simulink model "PI_with_st_pttracking"  (R2021a)
settings: Solver=VariableStepAuto  StartTime=0.0  StopTime=2500  RelTol=1e-3
libraries: simulink x4, pid_lib x4
settings Model: Creator=jessilbijou  LastModifiedBy=jessilbijou

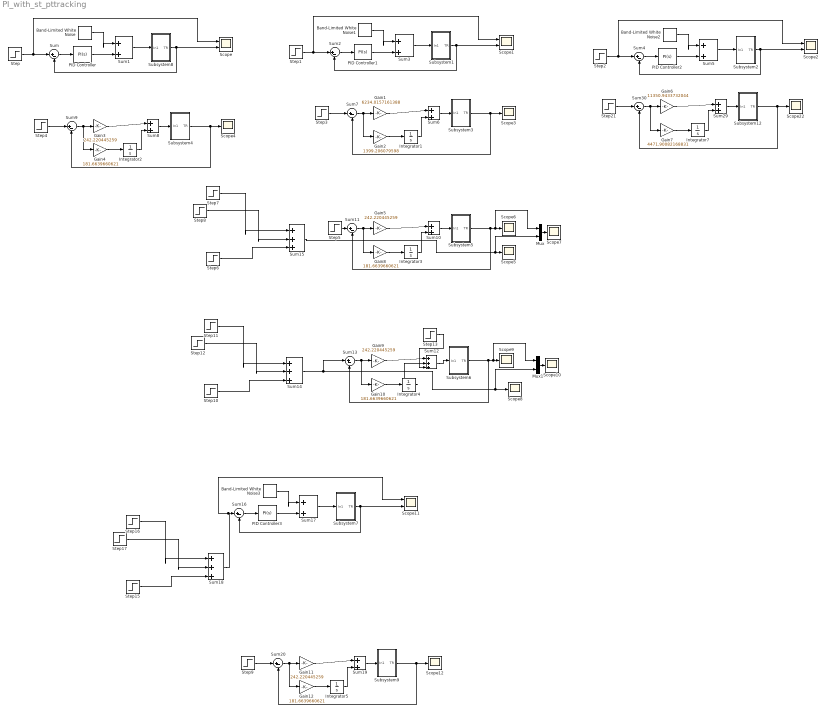
== system PI_with_st_pttracking ==
  Band-Limited White Noise{,1..3} (4 alike) : simulink/Sources/Band-Limited White Noise  Cov=[0.1]  Ts=0.1  seed=[23341]
  Gain1 : Gain  Gain=6234.0157161388
  Gain{4,8,10,12} (4 alike) : Gain  Gain=181.6639660621
  Gain{3,5,9,11} (4 alike) : Gain  Gain=242.220445259
  Gain2 : Gain  Gain=1399.206079598
  Gain6 : Gain  Gain=11350.9433732044
  Gain7 : Gain  Gain=4471.90082168831
  Integrator{1..5,7} (6 alike) : Integrator
  Mux : Mux  Inputs=2
  Mux1 : Mux  Inputs=2
  PID Controller : pid_lib/PID Controller  Controller=PI  Form=Parallel  TimeDomain=Continuous-time  UseExternalTs=off  SampleTime=-1  IntegratorMethod=Forward Euler  FilterMethod=Forward Euler  ControllerParametersSource=internal  P=242.220445259  I=181.6639660621  D=0  UseFilter=on  N=100  TunerSelectOption=Transfer Function Based (PID Tuner App)  InitialConditionSource=internal  InitialConditionForIntegrator=0  InitialConditionForFilter=0  DifferentiatorICPrevScaledInput=0  ExternalReset=none  TrackingMode=off  Kt=1  LimitOutput=off  SatLimitsSource=internal  UpperSaturationLimit=inf  LowerSaturationLimit=-inf  LinearizeAsGain=on  AntiWindupMode=none  Kb=1  POutMin=[]  POutMax=[]  IOutMin=[]  IOutMax=[]  DOutMin=[]  DOutMax=[]  NOutMin=[]  NOutMax=[]  SumOutMin=[]  SumOutMax=[]  SaturationOutMin=[]  SaturationOutMax=[]  PParamMin=[]  PParamMax=[]  IParamMin=[]  IParamMax=[]  DParamMin=[]  DParamMax=[]  NParamMin=[]  NParamMax=[]  KbParamMin=[]  KbParamMax=[]  KtParamMin=[]  KtParamMax=[]  KbOutMin=[]  KbOutMax=[]  KtOutMin=[]  KtOutMax=[]  IntegratorOutMin=[]  IntegratorOutMax=[]  FilterOutMin=[]  FilterOutMax=[]  SumI1OutMin=[]  SumI1OutMax=[]  SumI2OutMin=[]  SumI2OutMax=[]  SumI3OutMin=[]  SumI3OutMax=[]  SumI4OutMin=[]  SumI4OutMax=[]  SumDOutMin=[]  SumDOutMax=[]  DifferentiatorOutMin=[]  DifferentiatorOutMax=[]  FilterDiffOutCoefMin=[]  FilterDiffOutCoefMax=[]  ReciprocalOutMin=[]  ReciprocalOutMax=[]  SumDenOutMin=[]  SumDenOutMax=[]  SumNumOutMin=[]  SumNumOutMax=[]  DivideOutMin=[]  DivideOutMax=[]  UdiffTsProdOutMin=[]  UdiffTsProdOutMax=[]  NTsProdOutMin=[]  NTsProdOutMax=[]  UintegralTsProdOutMin=[]  UintegralTsProdOutMax=[]  UngainTsProdOutMin=[]  UngainTsProdOutMax=[]  IntegratorContinuousStateAttributes=''  IntegratorStateMustResolveToSignalObject=off  IntegratorRTWStateStorageClass=Auto  FilterContinuousStateAttributes=''  FilterStateMustResolveToSignalObject=off  FilterRTWStateStorageClass=Auto  ParallelPVariant=InternalParameters  IdealPVariant=Disabled  IVariant=InternalParameters  DVariant=Disabled  IntegratorVariant=Continuous  SatVariant=Disabled  AWVariant=Passthrough  PCopyVariant=Disabled  TRVariant=Disabled  FdbkBlocksVariant=Forward  IdealPFdbkVariant=Disabled  SatFdbkVariant=Disabled  DerivativeFilterVariant=Disabled  NVariant=Disabled  NCopyVariant=Disabled_SignalSpec  FilterICVariant=Disabled  IntegratorICVariant=InternalICs  ExternalResetVariant=Disabled  TRSumVariant=Passthrough  SumFdbkVariant=Disabled  SumVariant=Sum_PI  TsampFilterVariant=InternalTs  TsampNgainVariant=Passthrough  TsampIntegralVariant=Passthrough  ExternalSaturationOutDataTypeStr=Inherit: Same as second input
  PID Controller1 : pid_lib/PID Controller  Controller=PI  Form=Parallel  TimeDomain=Continuous-time  UseExternalTs=off  SampleTime=-1  IntegratorMethod=Forward Euler  FilterMethod=Forward Euler  ControllerParametersSource=internal  P=6234.0157161388  I=1399.206079598  D=0  UseFilter=on  N=100  TunerSelectOption=Transfer Function Based (PID Tuner App)  InitialConditionSource=internal  InitialConditionForIntegrator=0  InitialConditionForFilter=0  DifferentiatorICPrevScaledInput=0  ExternalReset=none  TrackingMode=off  Kt=1  LimitOutput=off  SatLimitsSource=internal  UpperSaturationLimit=inf  LowerSaturationLimit=-inf  LinearizeAsGain=on  AntiWindupMode=none  Kb=1  POutMin=[]  POutMax=[]  IOutMin=[]  IOutMax=[]  DOutMin=[]  DOutMax=[]  NOutMin=[]  NOutMax=[]  SumOutMin=[]  SumOutMax=[]  SaturationOutMin=[]  SaturationOutMax=[]  PParamMin=[]  PParamMax=[]  IParamMin=[]  IParamMax=[]  DParamMin=[]  DParamMax=[]  NParamMin=[]  NParamMax=[]  KbParamMin=[]  KbParamMax=[]  KtParamMin=[]  KtParamMax=[]  KbOutMin=[]  KbOutMax=[]  KtOutMin=[]  KtOutMax=[]  IntegratorOutMin=[]  IntegratorOutMax=[]  FilterOutMin=[]  FilterOutMax=[]  SumI1OutMin=[]  SumI1OutMax=[]  SumI2OutMin=[]  SumI2OutMax=[]  SumI3OutMin=[]  SumI3OutMax=[]  SumI4OutMin=[]  SumI4OutMax=[]  SumDOutMin=[]  SumDOutMax=[]  DifferentiatorOutMin=[]  DifferentiatorOutMax=[]  FilterDiffOutCoefMin=[]  FilterDiffOutCoefMax=[]  ReciprocalOutMin=[]  ReciprocalOutMax=[]  SumDenOutMin=[]  SumDenOutMax=[]  SumNumOutMin=[]  SumNumOutMax=[]  DivideOutMin=[]  DivideOutMax=[]  UdiffTsProdOutMin=[]  UdiffTsProdOutMax=[]  NTsProdOutMin=[]  NTsProdOutMax=[]  UintegralTsProdOutMin=[]  UintegralTsProdOutMax=[]  UngainTsProdOutMin=[]  UngainTsProdOutMax=[]  IntegratorContinuousStateAttributes=''  IntegratorStateMustResolveToSignalObject=off  IntegratorRTWStateStorageClass=Auto  FilterContinuousStateAttributes=''  FilterStateMustResolveToSignalObject=off  FilterRTWStateStorageClass=Auto  ParallelPVariant=InternalParameters  IdealPVariant=Disabled  IVariant=InternalParameters  DVariant=Disabled  IntegratorVariant=Continuous  SatVariant=Disabled  AWVariant=Passthrough  PCopyVariant=Disabled  TRVariant=Disabled  FdbkBlocksVariant=Forward  IdealPFdbkVariant=Disabled  SatFdbkVariant=Disabled  DerivativeFilterVariant=Disabled  NVariant=Disabled  NCopyVariant=Disabled_SignalSpec  FilterICVariant=Disabled  IntegratorICVariant=InternalICs  ExternalResetVariant=Disabled  TRSumVariant=Passthrough  SumFdbkVariant=Disabled  SumVariant=Sum_PI  TsampFilterVariant=InternalTs  TsampNgainVariant=Passthrough  TsampIntegralVariant=Passthrough  ExternalSaturationOutDataTypeStr=Inherit: Same as second input
  PID Controller2 : pid_lib/PID Controller  Controller=PI  Form=Parallel  TimeDomain=Continuous-time  UseExternalTs=off  SampleTime=-1  IntegratorMethod=Forward Euler  FilterMethod=Forward Euler  ControllerParametersSource=internal  P=11350.9433732044  I=4471.90082168831  D=0  UseFilter=on  N=100  TunerSelectOption=Transfer Function Based (PID Tuner App)  InitialConditionSource=internal  InitialConditionForIntegrator=0  InitialConditionForFilter=0  DifferentiatorICPrevScaledInput=0  ExternalReset=none  TrackingMode=off  Kt=1  LimitOutput=off  SatLimitsSource=internal  UpperSaturationLimit=inf  LowerSaturationLimit=-inf  LinearizeAsGain=on  AntiWindupMode=none  Kb=1  POutMin=[]  POutMax=[]  IOutMin=[]  IOutMax=[]  DOutMin=[]  DOutMax=[]  NOutMin=[]  NOutMax=[]  SumOutMin=[]  SumOutMax=[]  SaturationOutMin=[]  SaturationOutMax=[]  PParamMin=[]  PParamMax=[]  IParamMin=[]  IParamMax=[]  DParamMin=[]  DParamMax=[]  NParamMin=[]  NParamMax=[]  KbParamMin=[]  KbParamMax=[]  KtParamMin=[]  KtParamMax=[]  KbOutMin=[]  KbOutMax=[]  KtOutMin=[]  KtOutMax=[]  IntegratorOutMin=[]  IntegratorOutMax=[]  FilterOutMin=[]  FilterOutMax=[]  SumI1OutMin=[]  SumI1OutMax=[]  SumI2OutMin=[]  SumI2OutMax=[]  SumI3OutMin=[]  SumI3OutMax=[]  SumI4OutMin=[]  SumI4OutMax=[]  SumDOutMin=[]  SumDOutMax=[]  DifferentiatorOutMin=[]  DifferentiatorOutMax=[]  FilterDiffOutCoefMin=[]  FilterDiffOutCoefMax=[]  ReciprocalOutMin=[]  ReciprocalOutMax=[]  SumDenOutMin=[]  SumDenOutMax=[]  SumNumOutMin=[]  SumNumOutMax=[]  DivideOutMin=[]  DivideOutMax=[]  UdiffTsProdOutMin=[]  UdiffTsProdOutMax=[]  NTsProdOutMin=[]  NTsProdOutMax=[]  UintegralTsProdOutMin=[]  UintegralTsProdOutMax=[]  UngainTsProdOutMin=[]  UngainTsProdOutMax=[]  IntegratorContinuousStateAttributes=''  IntegratorStateMustResolveToSignalObject=off  IntegratorRTWStateStorageClass=Auto  FilterContinuousStateAttributes=''  FilterStateMustResolveToSignalObject=off  FilterRTWStateStorageClass=Auto  ParallelPVariant=InternalParameters  IdealPVariant=Disabled  IVariant=InternalParameters  DVariant=Disabled  IntegratorVariant=Continuous  SatVariant=Disabled  AWVariant=Passthrough  PCopyVariant=Disabled  TRVariant=Disabled  FdbkBlocksVariant=Forward  IdealPFdbkVariant=Disabled  SatFdbkVariant=Disabled  DerivativeFilterVariant=Disabled  NVariant=Disabled  NCopyVariant=Disabled_SignalSpec  FilterICVariant=Disabled  IntegratorICVariant=InternalICs  ExternalResetVariant=Disabled  TRSumVariant=Passthrough  SumFdbkVariant=Disabled  SumVariant=Sum_PI  TsampFilterVariant=InternalTs  TsampNgainVariant=Passthrough  TsampIntegralVariant=Passthrough  ExternalSaturationOutDataTypeStr=Inherit: Same as second input
  PID Controller3 : pid_lib/PID Controller  Controller=PI  Form=Parallel  TimeDomain=Continuous-time  UseExternalTs=off  SampleTime=-1  IntegratorMethod=Forward Euler  FilterMethod=Forward Euler  ControllerParametersSource=internal  P=242.220445259  I=181.6639660621  D=0  UseFilter=on  N=100  TunerSelectOption=Transfer Function Based (PID Tuner App)  InitialConditionSource=internal  InitialConditionForIntegrator=0  InitialConditionForFilter=0  DifferentiatorICPrevScaledInput=0  ExternalReset=none  TrackingMode=off  Kt=1  LimitOutput=off  SatLimitsSource=internal  UpperSaturationLimit=inf  LowerSaturationLimit=-inf  LinearizeAsGain=on  AntiWindupMode=none  Kb=1  POutMin=[]  POutMax=[]  IOutMin=[]  IOutMax=[]  DOutMin=[]  DOutMax=[]  NOutMin=[]  NOutMax=[]  SumOutMin=[]  SumOutMax=[]  SaturationOutMin=[]  SaturationOutMax=[]  PParamMin=[]  PParamMax=[]  IParamMin=[]  IParamMax=[]  DParamMin=[]  DParamMax=[]  NParamMin=[]  NParamMax=[]  KbParamMin=[]  KbParamMax=[]  KtParamMin=[]  KtParamMax=[]  KbOutMin=[]  KbOutMax=[]  KtOutMin=[]  KtOutMax=[]  IntegratorOutMin=[]  IntegratorOutMax=[]  FilterOutMin=[]  FilterOutMax=[]  SumI1OutMin=[]  SumI1OutMax=[]  SumI2OutMin=[]  SumI2OutMax=[]  SumI3OutMin=[]  SumI3OutMax=[]  SumI4OutMin=[]  SumI4OutMax=[]  SumDOutMin=[]  SumDOutMax=[]  DifferentiatorOutMin=[]  DifferentiatorOutMax=[]  FilterDiffOutCoefMin=[]  FilterDiffOutCoefMax=[]  ReciprocalOutMin=[]  ReciprocalOutMax=[]  SumDenOutMin=[]  SumDenOutMax=[]  SumNumOutMin=[]  SumNumOutMax=[]  DivideOutMin=[]  DivideOutMax=[]  UdiffTsProdOutMin=[]  UdiffTsProdOutMax=[]  NTsProdOutMin=[]  NTsProdOutMax=[]  UintegralTsProdOutMin=[]  UintegralTsProdOutMax=[]  UngainTsProdOutMin=[]  UngainTsProdOutMax=[]  IntegratorContinuousStateAttributes=''  IntegratorStateMustResolveToSignalObject=off  IntegratorRTWStateStorageClass=Auto  FilterContinuousStateAttributes=''  FilterStateMustResolveToSignalObject=off  FilterRTWStateStorageClass=Auto  ParallelPVariant=InternalParameters  IdealPVariant=Disabled  IVariant=InternalParameters  DVariant=Disabled  IntegratorVariant=Continuous  SatVariant=Disabled  AWVariant=Passthrough  PCopyVariant=Disabled  TRVariant=Disabled  FdbkBlocksVariant=Forward  IdealPFdbkVariant=Disabled  SatFdbkVariant=Disabled  DerivativeFilterVariant=Disabled  NVariant=Disabled  NCopyVariant=Disabled_SignalSpec  FilterICVariant=Disabled  IntegratorICVariant=InternalICs  ExternalResetVariant=Disabled  TRSumVariant=Passthrough  SumFdbkVariant=Disabled  SumVariant=Sum_PI  TsampFilterVariant=InternalTs  TsampNgainVariant=Passthrough  TsampIntegralVariant=Passthrough  ExternalSaturationOutDataTypeStr=Inherit: Same as second input
  Scope{,1..2,11} (4 alike) : Scope  NumInputPorts=2
  Scope{3..10,12,22} (10 alike) : Scope
  Step{,1..2,21} (4 alike) : Step  Time=0  Before=415  After=418  SampleTime=0
  Step10 : Step  Time=0  After=0  SampleTime=0
  Step{4..5,9,11} (4 alike) : Step  Time=100  Before=415  After=418  SampleTime=0
  Step{8,12..13,17} (4 alike) : Step  Time=700  After=-3  SampleTime=0
  Step15 : Step  Time=10  SampleTime=0
  Step16 : Step  Time=100  Before=415  After=417  SampleTime=0
  Step3 : Step  Time=0  Before=415  After=415.1  SampleTime=0
  Step6 : Step  Time=10  SampleTime=0
  Step7 : Step  Time=100  Before=415  After=417  SampleTime=0
  Subsystem1 : Subsystem
  Subsystem12 : Subsystem
  Subsystem2 : Subsystem
  Subsystem3 : Subsystem
  Subsystem4 : Subsystem
  Subsystem5 : Subsystem
  Subsystem6 : Subsystem
  Subsystem7 : Subsystem
  Subsystem8 : Subsystem
  Subsystem9 : Subsystem
  Sum{,2,4,7,9,11,13,16,20,30} (10 alike) : Sum  Inputs=|+-
  Sum{1,3,5..6,8,10,17,19,29} (9 alike) : Sum  Inputs=|++
  Sum{12,14..15,18} (4 alike) : Sum  Inputs=|+++
  wires:
  PID Controller1/1 -> Sum3/2
  Step1/1 -> Scope1/1, Sum2/1
  Band-Limited White Noise1/1 -> Sum3/1
  Sum2/1 -> PID Controller1/1
  Sum3/1 -> Subsystem1/1(In1)
  Subsystem1/1(TR) -> Sum2/2, Scope1/2
  PID Controller2/1 -> Sum5/2
  Step2/1 -> Scope2/1, Sum4/1
  Band-Limited White Noise2/1 -> Sum5/1
  Sum4/1 -> PID Controller2/1
  Sum5/1 -> Subsystem2/1(In1)
  Subsystem2/1(TR) -> Sum4/2, Scope2/2
  Gain7/1 -> Integrator7/1
  Gain6/1 -> Sum29/1
  Step21/1 -> Sum30/1
  Subsystem12/1(TR) -> Sum30/2, Scope22/1
  Sum30/1 -> Gain7/1, Gain6/1
  Sum29/1 -> Subsystem12/1(In1)
  Integrator7/1 -> Sum29/2
  PID Controller/1 -> Sum1/2
  Step/1 -> Scope/1, Sum/1
  Band-Limited White Noise/1 -> Sum1/1
  Sum/1 -> PID Controller/1
  Sum1/1 -> Subsystem8/1(In1)
  Subsystem8/1(TR) -> Sum/2, Scope/2
  Sum7/1 -> Gain2/1, Gain1/1
  Sum6/1 -> Subsystem3/1(In1)
  Gain1/1 -> Sum6/1
  Integrator1/1 -> Sum6/2
  Subsystem3/1(TR) -> Sum7/2, Scope3/1
  Step3/1 -> Sum7/1
  Gain2/1 -> Integrator1/1
  Sum9/1 -> Gain4/1, Gain3/1
  Sum8/1 -> Subsystem4/1(In1)
  Gain3/1 -> Sum8/1
  Integrator2/1 -> Sum8/2
  Subsystem4/1(TR) -> Sum9/2, Scope4/1
  Step4/1 -> Sum9/1
  Gain4/1 -> Integrator2/1
  Step8/1 -> Sum15/2
  Step7/1 -> Sum15/1
  Step6/1 -> Sum15/3
  Sum10/1 -> Subsystem5/1(In1)
  Subsystem5/1(TR) -> Sum11/2, Mux/1, Scope6/1
  Integrator3/1 -> Sum10/2
  Gain5/1 -> Sum10/1
  Sum11/1 -> Gain8/1, Gain5/1
  Gain8/1 -> Integrator3/1
  Step5/1 -> Sum11/1
  Sum15/1 -> Mux/2, Scope5/1
  Mux/1 -> Scope7/1
  Step12/1 -> Sum14/2
  Step11/1 -> Sum14/1
  Integrator4/1 -> Sum12/2
  Step10/1 -> Sum14/3
  Sum12/1 -> Subsystem6/1(In1)
  Sum14/1 -> Mux1/2, Scope8/1, Sum13/1
  Mux1/1 -> Scope10/1
  Subsystem6/1(TR) -> Sum13/2, Mux1/1, Scope9/1
  Gain10/1 -> Integrator4/1
  Sum13/1 -> Gain10/1, Gain9/1
  Gain9/1 -> Sum12/1
  Step13/1 -> Sum12/3
  Subsystem7/1(TR) -> Sum16/2, Scope11/2
  Band-Limited White Noise3/1 -> Sum17/1
  Sum18/1 -> Scope11/1, Sum16/1
  PID Controller3/1 -> Sum17/2
  Sum16/1 -> PID Controller3/1
  Sum17/1 -> Subsystem7/1(In1)
  Step15/1 -> Sum18/3
  Step17/1 -> Sum18/2
  Step16/1 -> Sum18/1
  Gain11/1 -> Sum19/1
  Sum19/1 -> Subsystem9/1(In1)
  Integrator5/1 -> Sum19/2
  Sum20/1 -> Gain12/1, Gain11/1
  Step9/1 -> Sum20/1
  Gain12/1 -> Integrator5/1
  Subsystem9/1(TR) -> Sum20/2, Scope12/1

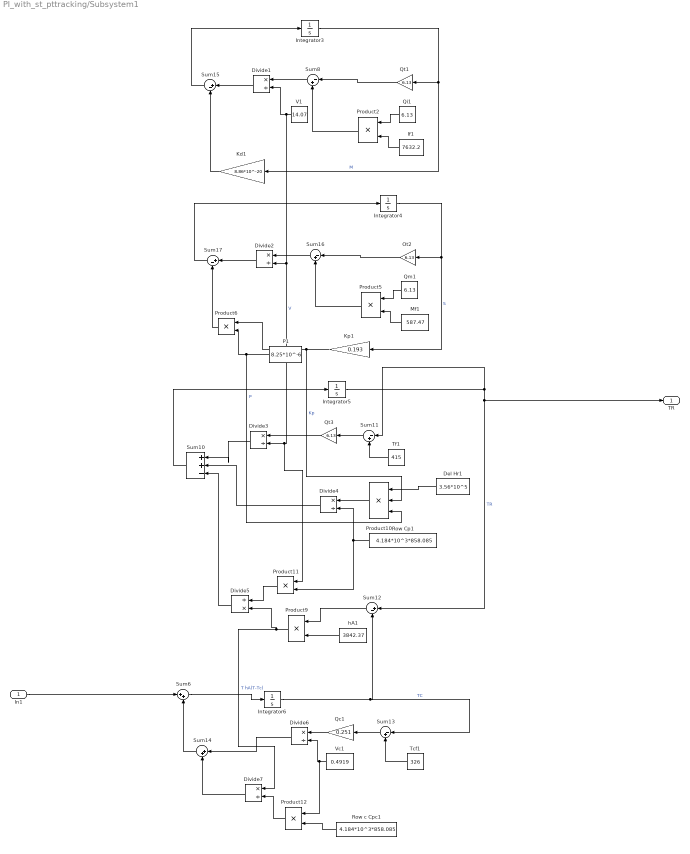
== system PI_with_st_pttracking/Subsystem1 ==
  In1 : Inport
  Del Hr1 : Constant  Value=3.56*10^5
  Divide{1..4,6..7} (6 alike) : Product  Inputs=*/
  Divide5 : Product  Inputs=/*
  If1 : Constant  Value=7632.2
  Integrator3 : Integrator  InitialCondition=7632.2
  Integrator4 : Integrator  InitialCondition=587.47
  Integrator5 : Integrator  InitialCondition=415
  Integrator6 : Integrator  InitialCondition=326
  Kd1 : Gain  Gain=8.86*10^-20
  Kp1 : Gain  Gain=0.193
  Mf1 : Constant  Value=587.47
  Ot2 : Gain  Gain=6.13
  P1 : Constant  Value=8.25*10^-6
  Product10 : Product  Inputs=3
  Product{2,5..6,9,11..12} (6 alike) : Product
  Qc1 : Gain  Gain=0.251
  Qi1 : Constant  Value=6.13
  Qm1 : Constant  Value=6.13
  Qt1 : Gain  Gain=6.13
  Qt3 : Gain  Gain=6.13
  Row Cp1 : Constant  Value=4.184*10^3*858.085
  Row c Cpc1 : Constant  Value=4.184*10^3*858.085
  Sum10 : Sum  Inputs=|++-
  Sum{8,11,13,16} (4 alike) : Sum  Inputs=|-+
  Sum12 : Sum  Inputs=|+-
  Sum14 : Sum  Inputs=|++
  Sum15 : Sum  Inputs=|+-
  Sum17 : Sum  Inputs=|+-
  Sum6 : Sum  Inputs=|++
  Tcf1 : Constant  Value=326
  Tf1 : Constant  Value=415
  V1 : Constant  Value=14.07
  Vc1 : Constant  Value=0.4919
  hA1 : Constant  Value=3842.37
  TR : Outport
  wires:
  Qm1/1 -> Product5/1
  Sum12/1 -> Product9/1
  Sum10/1 -> Integrator5/1
  Integrator5/1 -> TR/1, Sum12/1, Sum11/1  "TR"
  Ot2/1 -> Sum16/1
  Product11/1 -> Divide5/1
  Divide4/1 -> Sum10/2
  Sum16/1 -> Divide2/1
  Del Hr1/1 -> Product10/1
  Qi1/1 -> Product2/1
  Divide5/1 -> Sum10/3
  hA1/1 -> Product9/2
  Row c Cpc1/1 -> Product12/2
  Product10/1 -> Divide4/1
  Kd1/1 -> Sum15/2
  If1/1 -> Product2/2
  Divide3/1 -> Sum10/1
  Product6/1 -> Sum17/2
  Mf1/1 -> Product5/2
  Sum17/1 -> Integrator4/1
  Qt1/1 -> Sum8/1
  Kp1/1 -> Product6/1, Product10/2  "Kp"
  Tcf1/1 -> Sum13/2
  Integrator3/1 -> Kd1/1, Qt1/1  "M"
  Product9/1 -> Divide5/2, Divide7/1  "T hA(T-Tc)"
  Sum15/1 -> Integrator3/1
  Row Cp1/1 -> Product11/2, Divide4/2
  Sum11/1 -> Qt3/1
  Divide1/1 -> Sum15/1
  Product5/1 -> Sum16/2
  P1/1 -> Product6/2, Product10/3  "P"
  Vc1/1 -> Product12/1, Divide6/2
  Product2/1 -> Sum8/2
  V1/1 -> Product11/1, Divide3/2, Divide2/2, Divide1/2  "V"
  Sum8/1 -> Divide1/1
  Integrator4/1 -> Kp1/1, Ot2/1  "S"
  Divide6/1 -> Sum14/1
  Divide2/1 -> Sum17/1
  Divide7/1 -> Sum14/2
  Tf1/1 -> Sum11/2
  Qc1/1 -> Divide6/1
  Sum13/1 -> Qc1/1
  Product12/1 -> Divide7/2
  Integrator6/1 -> Sum13/1, Sum12/2  "TC"
  Qt3/1 -> Divide3/1
  Sum14/1 -> Sum6/2
  In1/1 -> Sum6/1
  Sum6/1 -> Integrator6/1

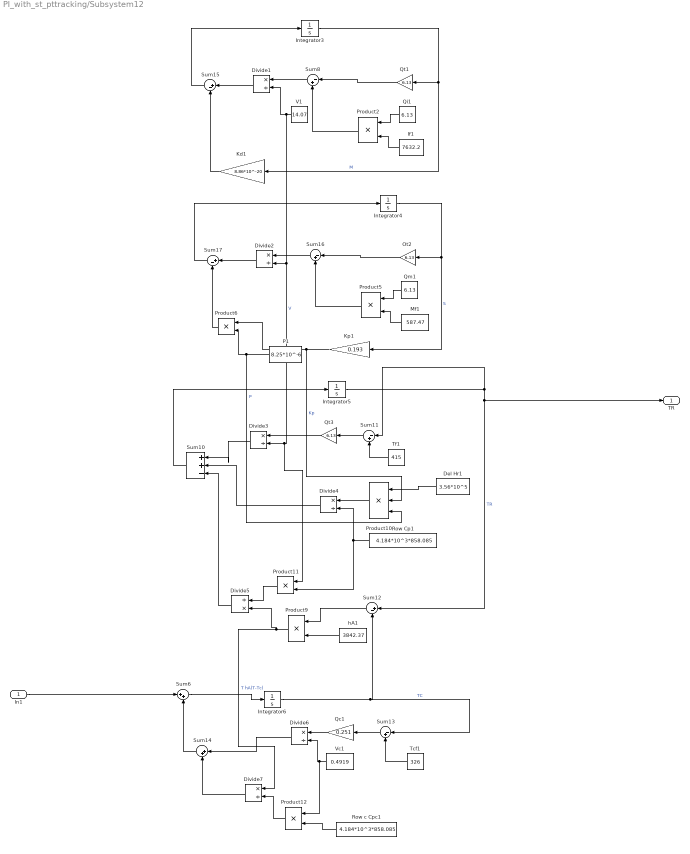
== system PI_with_st_pttracking/Subsystem12 ==
  In1 : Inport
  Del Hr1 : Constant  Value=3.56*10^5
  Divide{1..4,6..7} (6 alike) : Product  Inputs=*/
  Divide5 : Product  Inputs=/*
  If1 : Constant  Value=7632.2
  Integrator3 : Integrator  InitialCondition=7632.2
  Integrator4 : Integrator  InitialCondition=587.47
  Integrator5 : Integrator  InitialCondition=415
  Integrator6 : Integrator  InitialCondition=326
  Kd1 : Gain  Gain=8.86*10^-20
  Kp1 : Gain  Gain=0.193
  Mf1 : Constant  Value=587.47
  Ot2 : Gain  Gain=6.13
  P1 : Constant  Value=8.25*10^-6
  Product10 : Product  Inputs=3
  Product{2,5..6,9,11..12} (6 alike) : Product
  Qc1 : Gain  Gain=0.251
  Qi1 : Constant  Value=6.13
  Qm1 : Constant  Value=6.13
  Qt1 : Gain  Gain=6.13
  Qt3 : Gain  Gain=6.13
  Row Cp1 : Constant  Value=4.184*10^3*858.085
  Row c Cpc1 : Constant  Value=4.184*10^3*858.085
  Sum10 : Sum  Inputs=|++-
  Sum{8,11,13,16} (4 alike) : Sum  Inputs=|-+
  Sum12 : Sum  Inputs=|+-
  Sum14 : Sum  Inputs=|++
  Sum15 : Sum  Inputs=|+-
  Sum17 : Sum  Inputs=|+-
  Sum6 : Sum  Inputs=|++
  Tcf1 : Constant  Value=326
  Tf1 : Constant  Value=415
  V1 : Constant  Value=14.07
  Vc1 : Constant  Value=0.4919
  hA1 : Constant  Value=3842.37
  TR : Outport
  wires:
  Qm1/1 -> Product5/1
  Sum12/1 -> Product9/1
  Sum10/1 -> Integrator5/1
  Integrator5/1 -> TR/1, Sum12/1, Sum11/1  "TR"
  Ot2/1 -> Sum16/1
  Product11/1 -> Divide5/1
  Divide4/1 -> Sum10/2
  Sum16/1 -> Divide2/1
  Del Hr1/1 -> Product10/1
  Qi1/1 -> Product2/1
  Divide5/1 -> Sum10/3
  hA1/1 -> Product9/2
  Row c Cpc1/1 -> Product12/2
  Product10/1 -> Divide4/1
  Kd1/1 -> Sum15/2
  If1/1 -> Product2/2
  Divide3/1 -> Sum10/1
  Product6/1 -> Sum17/2
  Mf1/1 -> Product5/2
  Sum17/1 -> Integrator4/1
  Qt1/1 -> Sum8/1
  Kp1/1 -> Product6/1, Product10/2  "Kp"
  Tcf1/1 -> Sum13/2
  Integrator3/1 -> Kd1/1, Qt1/1  "M"
  Product9/1 -> Divide5/2, Divide7/1  "T hA(T-Tc)"
  Sum15/1 -> Integrator3/1
  Row Cp1/1 -> Product11/2, Divide4/2
  Sum11/1 -> Qt3/1
  Divide1/1 -> Sum15/1
  Product5/1 -> Sum16/2
  P1/1 -> Product6/2, Product10/3  "P"
  Vc1/1 -> Product12/1, Divide6/2
  Product2/1 -> Sum8/2
  V1/1 -> Product11/1, Divide3/2, Divide2/2, Divide1/2  "V"
  Sum8/1 -> Divide1/1
  Integrator4/1 -> Kp1/1, Ot2/1  "S"
  Divide6/1 -> Sum14/1
  Divide2/1 -> Sum17/1
  Divide7/1 -> Sum14/2
  Tf1/1 -> Sum11/2
  Qc1/1 -> Divide6/1
  Sum13/1 -> Qc1/1
  Product12/1 -> Divide7/2
  Integrator6/1 -> Sum13/1, Sum12/2  "TC"
  Qt3/1 -> Divide3/1
  Sum14/1 -> Sum6/2
  In1/1 -> Sum6/1
  Sum6/1 -> Integrator6/1

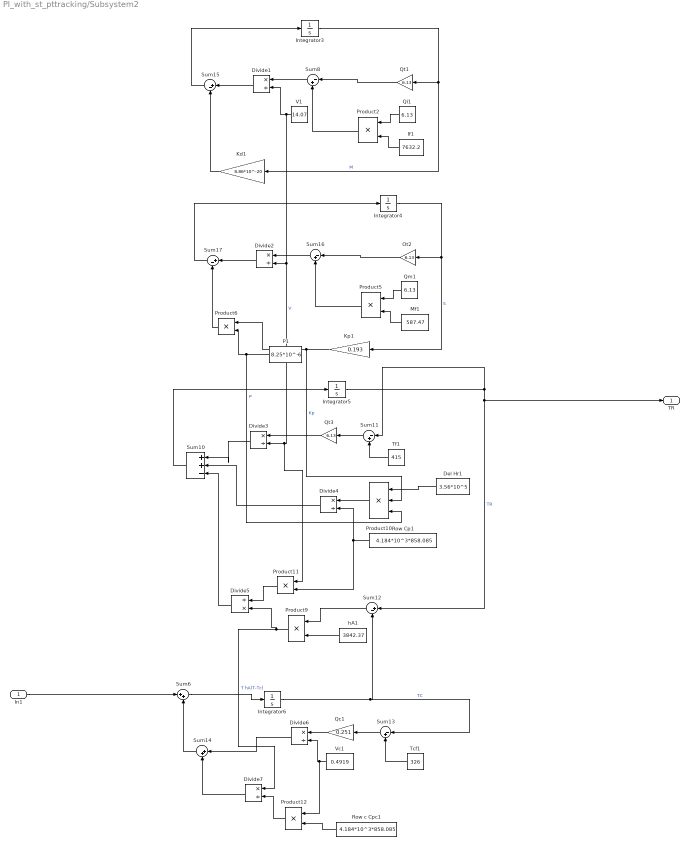
== system PI_with_st_pttracking/Subsystem2 ==
  In1 : Inport
  Del Hr1 : Constant  Value=3.56*10^5
  Divide{1..4,6..7} (6 alike) : Product  Inputs=*/
  Divide5 : Product  Inputs=/*
  If1 : Constant  Value=7632.2
  Integrator3 : Integrator  InitialCondition=7632.2
  Integrator4 : Integrator  InitialCondition=587.47
  Integrator5 : Integrator  InitialCondition=415
  Integrator6 : Integrator  InitialCondition=326
  Kd1 : Gain  Gain=8.86*10^-20
  Kp1 : Gain  Gain=0.193
  Mf1 : Constant  Value=587.47
  Ot2 : Gain  Gain=6.13
  P1 : Constant  Value=8.25*10^-6
  Product10 : Product  Inputs=3
  Product{2,5..6,9,11..12} (6 alike) : Product
  Qc1 : Gain  Gain=0.251
  Qi1 : Constant  Value=6.13
  Qm1 : Constant  Value=6.13
  Qt1 : Gain  Gain=6.13
  Qt3 : Gain  Gain=6.13
  Row Cp1 : Constant  Value=4.184*10^3*858.085
  Row c Cpc1 : Constant  Value=4.184*10^3*858.085
  Sum10 : Sum  Inputs=|++-
  Sum{8,11,13,16} (4 alike) : Sum  Inputs=|-+
  Sum12 : Sum  Inputs=|+-
  Sum14 : Sum  Inputs=|++
  Sum15 : Sum  Inputs=|+-
  Sum17 : Sum  Inputs=|+-
  Sum6 : Sum  Inputs=|++
  Tcf1 : Constant  Value=326
  Tf1 : Constant  Value=415
  V1 : Constant  Value=14.07
  Vc1 : Constant  Value=0.4919
  hA1 : Constant  Value=3842.37
  TR : Outport
  wires:
  Qm1/1 -> Product5/1
  Sum12/1 -> Product9/1
  Sum10/1 -> Integrator5/1
  Integrator5/1 -> TR/1, Sum12/1, Sum11/1  "TR"
  Ot2/1 -> Sum16/1
  Product11/1 -> Divide5/1
  Divide4/1 -> Sum10/2
  Sum16/1 -> Divide2/1
  Del Hr1/1 -> Product10/1
  Qi1/1 -> Product2/1
  Divide5/1 -> Sum10/3
  hA1/1 -> Product9/2
  Row c Cpc1/1 -> Product12/2
  Product10/1 -> Divide4/1
  Kd1/1 -> Sum15/2
  If1/1 -> Product2/2
  Divide3/1 -> Sum10/1
  Product6/1 -> Sum17/2
  Mf1/1 -> Product5/2
  Sum17/1 -> Integrator4/1
  Qt1/1 -> Sum8/1
  Kp1/1 -> Product6/1, Product10/2  "Kp"
  Tcf1/1 -> Sum13/2
  Integrator3/1 -> Kd1/1, Qt1/1  "M"
  Product9/1 -> Divide5/2, Divide7/1  "T hA(T-Tc)"
  Sum15/1 -> Integrator3/1
  Row Cp1/1 -> Product11/2, Divide4/2
  Sum11/1 -> Qt3/1
  Divide1/1 -> Sum15/1
  Product5/1 -> Sum16/2
  P1/1 -> Product6/2, Product10/3  "P"
  Vc1/1 -> Product12/1, Divide6/2
  Product2/1 -> Sum8/2
  V1/1 -> Product11/1, Divide3/2, Divide2/2, Divide1/2  "V"
  Sum8/1 -> Divide1/1
  Integrator4/1 -> Kp1/1, Ot2/1  "S"
  Divide6/1 -> Sum14/1
  Divide2/1 -> Sum17/1
  Divide7/1 -> Sum14/2
  Tf1/1 -> Sum11/2
  Qc1/1 -> Divide6/1
  Sum13/1 -> Qc1/1
  Product12/1 -> Divide7/2
  Integrator6/1 -> Sum13/1, Sum12/2  "TC"
  Qt3/1 -> Divide3/1
  Sum14/1 -> Sum6/2
  In1/1 -> Sum6/1
  Sum6/1 -> Integrator6/1

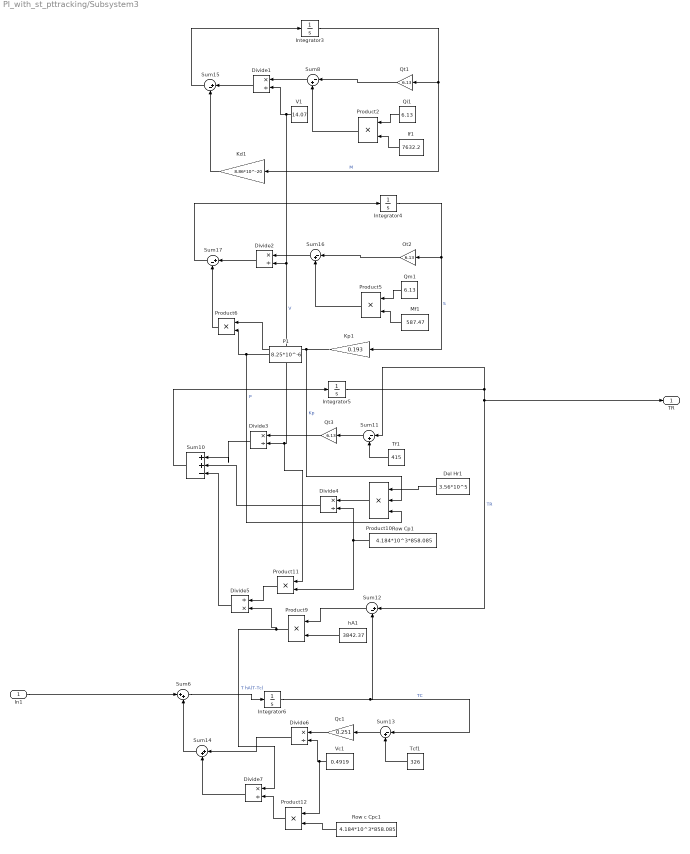
== system PI_with_st_pttracking/Subsystem3 ==
  In1 : Inport
  Del Hr1 : Constant  Value=3.56*10^5
  Divide{1..4,6..7} (6 alike) : Product  Inputs=*/
  Divide5 : Product  Inputs=/*
  If1 : Constant  Value=7632.2
  Integrator3 : Integrator  InitialCondition=7632.2
  Integrator4 : Integrator  InitialCondition=587.47
  Integrator5 : Integrator  InitialCondition=415
  Integrator6 : Integrator  InitialCondition=326
  Kd1 : Gain  Gain=8.86*10^-20
  Kp1 : Gain  Gain=0.193
  Mf1 : Constant  Value=587.47
  Ot2 : Gain  Gain=6.13
  P1 : Constant  Value=8.25*10^-6
  Product10 : Product  Inputs=3
  Product{2,5..6,9,11..12} (6 alike) : Product
  Qc1 : Gain  Gain=0.251
  Qi1 : Constant  Value=6.13
  Qm1 : Constant  Value=6.13
  Qt1 : Gain  Gain=6.13
  Qt3 : Gain  Gain=6.13
  Row Cp1 : Constant  Value=4.184*10^3*858.085
  Row c Cpc1 : Constant  Value=4.184*10^3*858.085
  Sum10 : Sum  Inputs=|++-
  Sum{8,11,13,16} (4 alike) : Sum  Inputs=|-+
  Sum12 : Sum  Inputs=|+-
  Sum14 : Sum  Inputs=|++
  Sum15 : Sum  Inputs=|+-
  Sum17 : Sum  Inputs=|+-
  Sum6 : Sum  Inputs=|++
  Tcf1 : Constant  Value=326
  Tf1 : Constant  Value=415
  V1 : Constant  Value=14.07
  Vc1 : Constant  Value=0.4919
  hA1 : Constant  Value=3842.37
  TR : Outport
  wires:
  Qm1/1 -> Product5/1
  Sum12/1 -> Product9/1
  Sum10/1 -> Integrator5/1
  Integrator5/1 -> TR/1, Sum12/1, Sum11/1  "TR"
  Ot2/1 -> Sum16/1
  Product11/1 -> Divide5/1
  Divide4/1 -> Sum10/2
  Sum16/1 -> Divide2/1
  Del Hr1/1 -> Product10/1
  Qi1/1 -> Product2/1
  Divide5/1 -> Sum10/3
  hA1/1 -> Product9/2
  Row c Cpc1/1 -> Product12/2
  Product10/1 -> Divide4/1
  Kd1/1 -> Sum15/2
  If1/1 -> Product2/2
  Divide3/1 -> Sum10/1
  Product6/1 -> Sum17/2
  Mf1/1 -> Product5/2
  Sum17/1 -> Integrator4/1
  Qt1/1 -> Sum8/1
  Kp1/1 -> Product6/1, Product10/2  "Kp"
  Tcf1/1 -> Sum13/2
  Integrator3/1 -> Kd1/1, Qt1/1  "M"
  Product9/1 -> Divide5/2, Divide7/1  "T hA(T-Tc)"
  Sum15/1 -> Integrator3/1
  Row Cp1/1 -> Product11/2, Divide4/2
  Sum11/1 -> Qt3/1
  Divide1/1 -> Sum15/1
  Product5/1 -> Sum16/2
  P1/1 -> Product6/2, Product10/3  "P"
  Vc1/1 -> Product12/1, Divide6/2
  Product2/1 -> Sum8/2
  V1/1 -> Product11/1, Divide3/2, Divide2/2, Divide1/2  "V"
  Sum8/1 -> Divide1/1
  Integrator4/1 -> Kp1/1, Ot2/1  "S"
  Divide6/1 -> Sum14/1
  Divide2/1 -> Sum17/1
  Divide7/1 -> Sum14/2
  Tf1/1 -> Sum11/2
  Qc1/1 -> Divide6/1
  Sum13/1 -> Qc1/1
  Product12/1 -> Divide7/2
  Integrator6/1 -> Sum13/1, Sum12/2  "TC"
  Qt3/1 -> Divide3/1
  Sum14/1 -> Sum6/2
  In1/1 -> Sum6/1
  Sum6/1 -> Integrator6/1

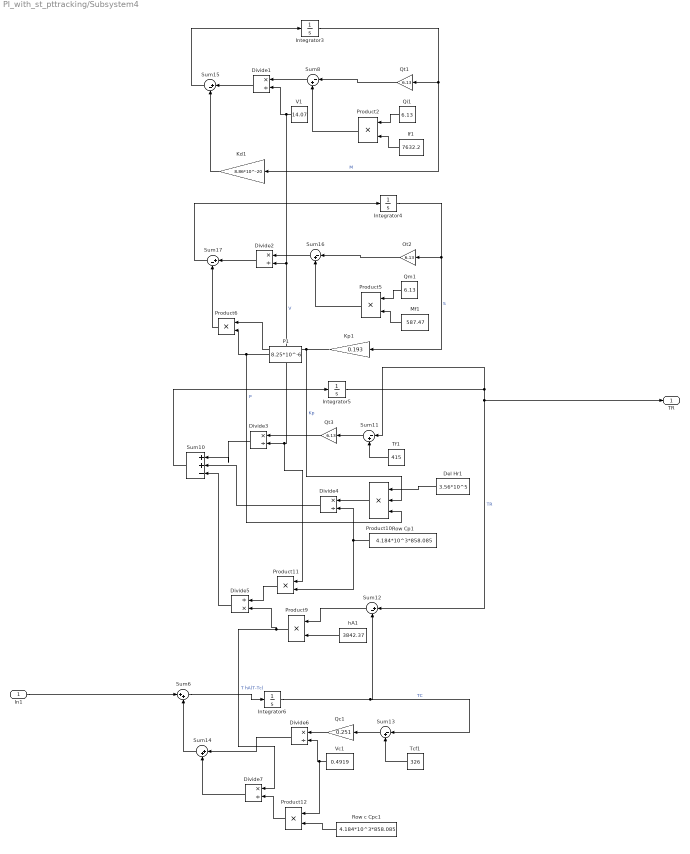
== system PI_with_st_pttracking/Subsystem4 ==
  In1 : Inport
  Del Hr1 : Constant  Value=3.56*10^5
  Divide{1..4,6..7} (6 alike) : Product  Inputs=*/
  Divide5 : Product  Inputs=/*
  If1 : Constant  Value=7632.2
  Integrator3 : Integrator  InitialCondition=7632.2
  Integrator4 : Integrator  InitialCondition=587.47
  Integrator5 : Integrator  InitialCondition=415
  Integrator6 : Integrator  InitialCondition=326
  Kd1 : Gain  Gain=8.86*10^-20
  Kp1 : Gain  Gain=0.193
  Mf1 : Constant  Value=587.47
  Ot2 : Gain  Gain=6.13
  P1 : Constant  Value=8.25*10^-6
  Product10 : Product  Inputs=3
  Product{2,5..6,9,11..12} (6 alike) : Product
  Qc1 : Gain  Gain=0.251
  Qi1 : Constant  Value=6.13
  Qm1 : Constant  Value=6.13
  Qt1 : Gain  Gain=6.13
  Qt3 : Gain  Gain=6.13
  Row Cp1 : Constant  Value=4.184*10^3*858.085
  Row c Cpc1 : Constant  Value=4.184*10^3*858.085
  Sum10 : Sum  Inputs=|++-
  Sum{8,11,13,16} (4 alike) : Sum  Inputs=|-+
  Sum12 : Sum  Inputs=|+-
  Sum14 : Sum  Inputs=|++
  Sum15 : Sum  Inputs=|+-
  Sum17 : Sum  Inputs=|+-
  Sum6 : Sum  Inputs=|++
  Tcf1 : Constant  Value=326
  Tf1 : Constant  Value=415
  V1 : Constant  Value=14.07
  Vc1 : Constant  Value=0.4919
  hA1 : Constant  Value=3842.37
  TR : Outport
  wires:
  Qm1/1 -> Product5/1
  Sum12/1 -> Product9/1
  Sum10/1 -> Integrator5/1
  Integrator5/1 -> TR/1, Sum12/1, Sum11/1  "TR"
  Ot2/1 -> Sum16/1
  Product11/1 -> Divide5/1
  Divide4/1 -> Sum10/2
  Sum16/1 -> Divide2/1
  Del Hr1/1 -> Product10/1
  Qi1/1 -> Product2/1
  Divide5/1 -> Sum10/3
  hA1/1 -> Product9/2
  Row c Cpc1/1 -> Product12/2
  Product10/1 -> Divide4/1
  Kd1/1 -> Sum15/2
  If1/1 -> Product2/2
  Divide3/1 -> Sum10/1
  Product6/1 -> Sum17/2
  Mf1/1 -> Product5/2
  Sum17/1 -> Integrator4/1
  Qt1/1 -> Sum8/1
  Kp1/1 -> Product6/1, Product10/2  "Kp"
  Tcf1/1 -> Sum13/2
  Integrator3/1 -> Kd1/1, Qt1/1  "M"
  Product9/1 -> Divide5/2, Divide7/1  "T hA(T-Tc)"
  Sum15/1 -> Integrator3/1
  Row Cp1/1 -> Product11/2, Divide4/2
  Sum11/1 -> Qt3/1
  Divide1/1 -> Sum15/1
  Product5/1 -> Sum16/2
  P1/1 -> Product6/2, Product10/3  "P"
  Vc1/1 -> Product12/1, Divide6/2
  Product2/1 -> Sum8/2
  V1/1 -> Product11/1, Divide3/2, Divide2/2, Divide1/2  "V"
  Sum8/1 -> Divide1/1
  Integrator4/1 -> Kp1/1, Ot2/1  "S"
  Divide6/1 -> Sum14/1
  Divide2/1 -> Sum17/1
  Divide7/1 -> Sum14/2
  Tf1/1 -> Sum11/2
  Qc1/1 -> Divide6/1
  Sum13/1 -> Qc1/1
  Product12/1 -> Divide7/2
  Integrator6/1 -> Sum13/1, Sum12/2  "TC"
  Qt3/1 -> Divide3/1
  Sum14/1 -> Sum6/2
  In1/1 -> Sum6/1
  Sum6/1 -> Integrator6/1

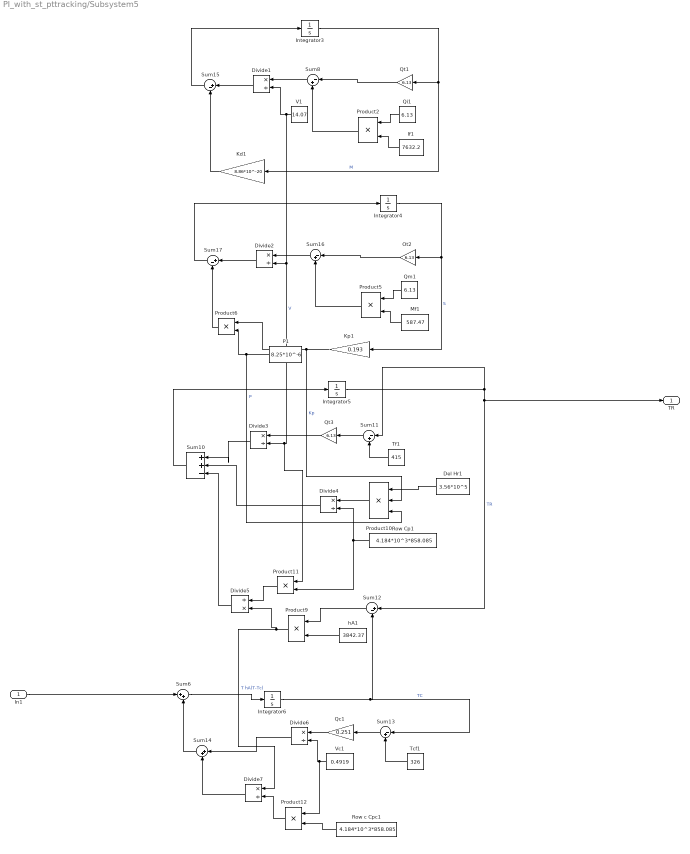
== system PI_with_st_pttracking/Subsystem5 ==
  In1 : Inport
  Del Hr1 : Constant  Value=3.56*10^5
  Divide{1..4,6..7} (6 alike) : Product  Inputs=*/
  Divide5 : Product  Inputs=/*
  If1 : Constant  Value=7632.2
  Integrator3 : Integrator  InitialCondition=7632.2
  Integrator4 : Integrator  InitialCondition=587.47
  Integrator5 : Integrator  InitialCondition=415
  Integrator6 : Integrator  InitialCondition=326
  Kd1 : Gain  Gain=8.86*10^-20
  Kp1 : Gain  Gain=0.193
  Mf1 : Constant  Value=587.47
  Ot2 : Gain  Gain=6.13
  P1 : Constant  Value=8.25*10^-6
  Product10 : Product  Inputs=3
  Product{2,5..6,9,11..12} (6 alike) : Product
  Qc1 : Gain  Gain=0.251
  Qi1 : Constant  Value=6.13
  Qm1 : Constant  Value=6.13
  Qt1 : Gain  Gain=6.13
  Qt3 : Gain  Gain=6.13
  Row Cp1 : Constant  Value=4.184*10^3*858.085
  Row c Cpc1 : Constant  Value=4.184*10^3*858.085
  Sum10 : Sum  Inputs=|++-
  Sum{8,11,13,16} (4 alike) : Sum  Inputs=|-+
  Sum12 : Sum  Inputs=|+-
  Sum14 : Sum  Inputs=|++
  Sum15 : Sum  Inputs=|+-
  Sum17 : Sum  Inputs=|+-
  Sum6 : Sum  Inputs=|++
  Tcf1 : Constant  Value=326
  Tf1 : Constant  Value=415
  V1 : Constant  Value=14.07
  Vc1 : Constant  Value=0.4919
  hA1 : Constant  Value=3842.37
  TR : Outport
  wires:
  Qm1/1 -> Product5/1
  Sum12/1 -> Product9/1
  Sum10/1 -> Integrator5/1
  Integrator5/1 -> TR/1, Sum12/1, Sum11/1  "TR"
  Ot2/1 -> Sum16/1
  Product11/1 -> Divide5/1
  Divide4/1 -> Sum10/2
  Sum16/1 -> Divide2/1
  Del Hr1/1 -> Product10/1
  Qi1/1 -> Product2/1
  Divide5/1 -> Sum10/3
  hA1/1 -> Product9/2
  Row c Cpc1/1 -> Product12/2
  Product10/1 -> Divide4/1
  Kd1/1 -> Sum15/2
  If1/1 -> Product2/2
  Divide3/1 -> Sum10/1
  Product6/1 -> Sum17/2
  Mf1/1 -> Product5/2
  Sum17/1 -> Integrator4/1
  Qt1/1 -> Sum8/1
  Kp1/1 -> Product6/1, Product10/2  "Kp"
  Tcf1/1 -> Sum13/2
  Integrator3/1 -> Kd1/1, Qt1/1  "M"
  Product9/1 -> Divide5/2, Divide7/1  "T hA(T-Tc)"
  Sum15/1 -> Integrator3/1
  Row Cp1/1 -> Product11/2, Divide4/2
  Sum11/1 -> Qt3/1
  Divide1/1 -> Sum15/1
  Product5/1 -> Sum16/2
  P1/1 -> Product6/2, Product10/3  "P"
  Vc1/1 -> Product12/1, Divide6/2
  Product2/1 -> Sum8/2
  V1/1 -> Product11/1, Divide3/2, Divide2/2, Divide1/2  "V"
  Sum8/1 -> Divide1/1
  Integrator4/1 -> Kp1/1, Ot2/1  "S"
  Divide6/1 -> Sum14/1
  Divide2/1 -> Sum17/1
  Divide7/1 -> Sum14/2
  Tf1/1 -> Sum11/2
  Qc1/1 -> Divide6/1
  Sum13/1 -> Qc1/1
  Product12/1 -> Divide7/2
  Integrator6/1 -> Sum13/1, Sum12/2  "TC"
  Qt3/1 -> Divide3/1
  Sum14/1 -> Sum6/2
  In1/1 -> Sum6/1
  Sum6/1 -> Integrator6/1

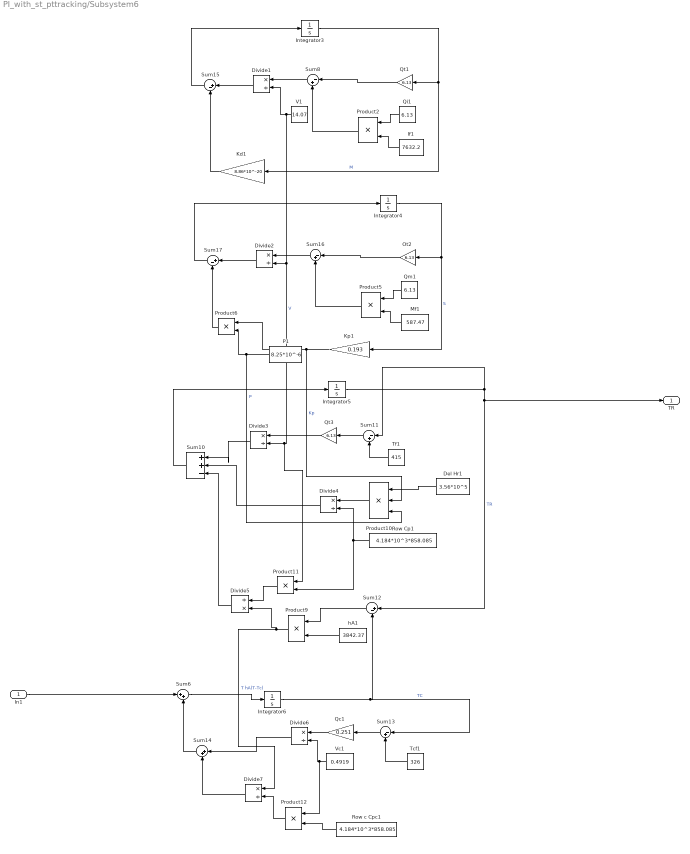
== system PI_with_st_pttracking/Subsystem6 ==
  In1 : Inport
  Del Hr1 : Constant  Value=3.56*10^5
  Divide{1..4,6..7} (6 alike) : Product  Inputs=*/
  Divide5 : Product  Inputs=/*
  If1 : Constant  Value=7632.2
  Integrator3 : Integrator  InitialCondition=7632.2
  Integrator4 : Integrator  InitialCondition=587.47
  Integrator5 : Integrator  InitialCondition=415
  Integrator6 : Integrator  InitialCondition=326
  Kd1 : Gain  Gain=8.86*10^-20
  Kp1 : Gain  Gain=0.193
  Mf1 : Constant  Value=587.47
  Ot2 : Gain  Gain=6.13
  P1 : Constant  Value=8.25*10^-6
  Product10 : Product  Inputs=3
  Product{2,5..6,9,11..12} (6 alike) : Product
  Qc1 : Gain  Gain=0.251
  Qi1 : Constant  Value=6.13
  Qm1 : Constant  Value=6.13
  Qt1 : Gain  Gain=6.13
  Qt3 : Gain  Gain=6.13
  Row Cp1 : Constant  Value=4.184*10^3*858.085
  Row c Cpc1 : Constant  Value=4.184*10^3*858.085
  Sum10 : Sum  Inputs=|++-
  Sum{8,11,13,16} (4 alike) : Sum  Inputs=|-+
  Sum12 : Sum  Inputs=|+-
  Sum14 : Sum  Inputs=|++
  Sum15 : Sum  Inputs=|+-
  Sum17 : Sum  Inputs=|+-
  Sum6 : Sum  Inputs=|++
  Tcf1 : Constant  Value=326
  Tf1 : Constant  Value=415
  V1 : Constant  Value=14.07
  Vc1 : Constant  Value=0.4919
  hA1 : Constant  Value=3842.37
  TR : Outport
  wires:
  Qm1/1 -> Product5/1
  Sum12/1 -> Product9/1
  Sum10/1 -> Integrator5/1
  Integrator5/1 -> TR/1, Sum12/1, Sum11/1  "TR"
  Ot2/1 -> Sum16/1
  Product11/1 -> Divide5/1
  Divide4/1 -> Sum10/2
  Sum16/1 -> Divide2/1
  Del Hr1/1 -> Product10/1
  Qi1/1 -> Product2/1
  Divide5/1 -> Sum10/3
  hA1/1 -> Product9/2
  Row c Cpc1/1 -> Product12/2
  Product10/1 -> Divide4/1
  Kd1/1 -> Sum15/2
  If1/1 -> Product2/2
  Divide3/1 -> Sum10/1
  Product6/1 -> Sum17/2
  Mf1/1 -> Product5/2
  Sum17/1 -> Integrator4/1
  Qt1/1 -> Sum8/1
  Kp1/1 -> Product6/1, Product10/2  "Kp"
  Tcf1/1 -> Sum13/2
  Integrator3/1 -> Kd1/1, Qt1/1  "M"
  Product9/1 -> Divide5/2, Divide7/1  "T hA(T-Tc)"
  Sum15/1 -> Integrator3/1
  Row Cp1/1 -> Product11/2, Divide4/2
  Sum11/1 -> Qt3/1
  Divide1/1 -> Sum15/1
  Product5/1 -> Sum16/2
  P1/1 -> Product6/2, Product10/3  "P"
  Vc1/1 -> Product12/1, Divide6/2
  Product2/1 -> Sum8/2
  V1/1 -> Product11/1, Divide3/2, Divide2/2, Divide1/2  "V"
  Sum8/1 -> Divide1/1
  Integrator4/1 -> Kp1/1, Ot2/1  "S"
  Divide6/1 -> Sum14/1
  Divide2/1 -> Sum17/1
  Divide7/1 -> Sum14/2
  Tf1/1 -> Sum11/2
  Qc1/1 -> Divide6/1
  Sum13/1 -> Qc1/1
  Product12/1 -> Divide7/2
  Integrator6/1 -> Sum13/1, Sum12/2  "TC"
  Qt3/1 -> Divide3/1
  Sum14/1 -> Sum6/2
  In1/1 -> Sum6/1
  Sum6/1 -> Integrator6/1

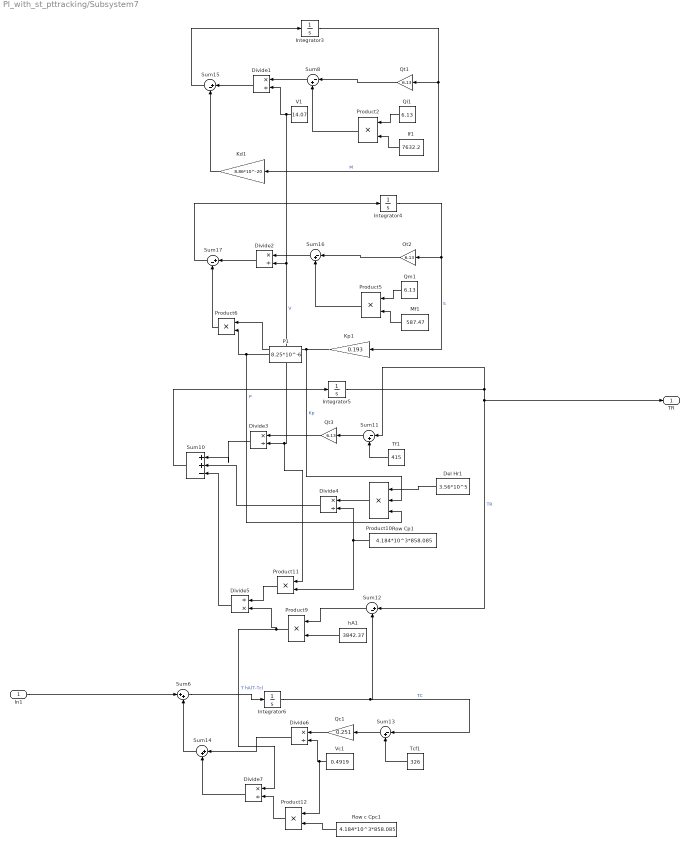
== system PI_with_st_pttracking/Subsystem7 ==
  In1 : Inport
  Del Hr1 : Constant  Value=3.56*10^5
  Divide{1..4,6..7} (6 alike) : Product  Inputs=*/
  Divide5 : Product  Inputs=/*
  If1 : Constant  Value=7632.2
  Integrator3 : Integrator  InitialCondition=7632.2
  Integrator4 : Integrator  InitialCondition=587.47
  Integrator5 : Integrator  InitialCondition=415
  Integrator6 : Integrator  InitialCondition=326
  Kd1 : Gain  Gain=8.86*10^-20
  Kp1 : Gain  Gain=0.193
  Mf1 : Constant  Value=587.47
  Ot2 : Gain  Gain=6.13
  P1 : Constant  Value=8.25*10^-6
  Product10 : Product  Inputs=3
  Product{2,5..6,9,11..12} (6 alike) : Product
  Qc1 : Gain  Gain=0.251
  Qi1 : Constant  Value=6.13
  Qm1 : Constant  Value=6.13
  Qt1 : Gain  Gain=6.13
  Qt3 : Gain  Gain=6.13
  Row Cp1 : Constant  Value=4.184*10^3*858.085
  Row c Cpc1 : Constant  Value=4.184*10^3*858.085
  Sum10 : Sum  Inputs=|++-
  Sum{8,11,13,16} (4 alike) : Sum  Inputs=|-+
  Sum12 : Sum  Inputs=|+-
  Sum14 : Sum  Inputs=|++
  Sum15 : Sum  Inputs=|+-
  Sum17 : Sum  Inputs=|+-
  Sum6 : Sum  Inputs=|++
  Tcf1 : Constant  Value=326
  Tf1 : Constant  Value=415
  V1 : Constant  Value=14.07
  Vc1 : Constant  Value=0.4919
  hA1 : Constant  Value=3842.37
  TR : Outport
  wires:
  Qm1/1 -> Product5/1
  Sum12/1 -> Product9/1
  Sum10/1 -> Integrator5/1
  Integrator5/1 -> TR/1, Sum12/1, Sum11/1  "TR"
  Ot2/1 -> Sum16/1
  Product11/1 -> Divide5/1
  Divide4/1 -> Sum10/2
  Sum16/1 -> Divide2/1
  Del Hr1/1 -> Product10/1
  Qi1/1 -> Product2/1
  Divide5/1 -> Sum10/3
  hA1/1 -> Product9/2
  Row c Cpc1/1 -> Product12/2
  Product10/1 -> Divide4/1
  Kd1/1 -> Sum15/2
  If1/1 -> Product2/2
  Divide3/1 -> Sum10/1
  Product6/1 -> Sum17/2
  Mf1/1 -> Product5/2
  Sum17/1 -> Integrator4/1
  Qt1/1 -> Sum8/1
  Kp1/1 -> Product6/1, Product10/2  "Kp"
  Tcf1/1 -> Sum13/2
  Integrator3/1 -> Kd1/1, Qt1/1  "M"
  Product9/1 -> Divide5/2, Divide7/1  "T hA(T-Tc)"
  Sum15/1 -> Integrator3/1
  Row Cp1/1 -> Product11/2, Divide4/2
  Sum11/1 -> Qt3/1
  Divide1/1 -> Sum15/1
  Product5/1 -> Sum16/2
  P1/1 -> Product6/2, Product10/3  "P"
  Vc1/1 -> Product12/1, Divide6/2
  Product2/1 -> Sum8/2
  V1/1 -> Product11/1, Divide3/2, Divide2/2, Divide1/2  "V"
  Sum8/1 -> Divide1/1
  Integrator4/1 -> Kp1/1, Ot2/1  "S"
  Divide6/1 -> Sum14/1
  Divide2/1 -> Sum17/1
  Divide7/1 -> Sum14/2
  Tf1/1 -> Sum11/2
  Qc1/1 -> Divide6/1
  Sum13/1 -> Qc1/1
  Product12/1 -> Divide7/2
  Integrator6/1 -> Sum13/1, Sum12/2  "TC"
  Qt3/1 -> Divide3/1
  Sum14/1 -> Sum6/2
  In1/1 -> Sum6/1
  Sum6/1 -> Integrator6/1

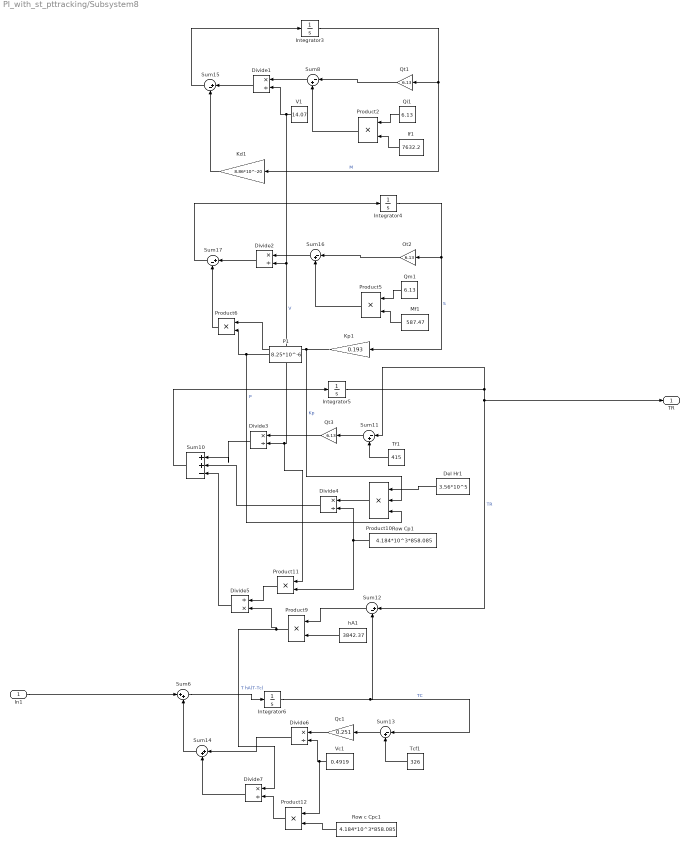
== system PI_with_st_pttracking/Subsystem8 ==
  In1 : Inport
  Del Hr1 : Constant  Value=3.56*10^5
  Divide{1..4,6..7} (6 alike) : Product  Inputs=*/
  Divide5 : Product  Inputs=/*
  If1 : Constant  Value=7632.2
  Integrator3 : Integrator  InitialCondition=7632.2
  Integrator4 : Integrator  InitialCondition=587.47
  Integrator5 : Integrator  InitialCondition=415
  Integrator6 : Integrator  InitialCondition=326
  Kd1 : Gain  Gain=8.86*10^-20
  Kp1 : Gain  Gain=0.193
  Mf1 : Constant  Value=587.47
  Ot2 : Gain  Gain=6.13
  P1 : Constant  Value=8.25*10^-6
  Product10 : Product  Inputs=3
  Product{2,5..6,9,11..12} (6 alike) : Product
  Qc1 : Gain  Gain=0.251
  Qi1 : Constant  Value=6.13
  Qm1 : Constant  Value=6.13
  Qt1 : Gain  Gain=6.13
  Qt3 : Gain  Gain=6.13
  Row Cp1 : Constant  Value=4.184*10^3*858.085
  Row c Cpc1 : Constant  Value=4.184*10^3*858.085
  Sum10 : Sum  Inputs=|++-
  Sum{8,11,13,16} (4 alike) : Sum  Inputs=|-+
  Sum12 : Sum  Inputs=|+-
  Sum14 : Sum  Inputs=|++
  Sum15 : Sum  Inputs=|+-
  Sum17 : Sum  Inputs=|+-
  Sum6 : Sum  Inputs=|++
  Tcf1 : Constant  Value=326
  Tf1 : Constant  Value=415
  V1 : Constant  Value=14.07
  Vc1 : Constant  Value=0.4919
  hA1 : Constant  Value=3842.37
  TR : Outport
  wires:
  Qm1/1 -> Product5/1
  Sum12/1 -> Product9/1
  Sum10/1 -> Integrator5/1
  Integrator5/1 -> TR/1, Sum12/1, Sum11/1  "TR"
  Ot2/1 -> Sum16/1
  Product11/1 -> Divide5/1
  Divide4/1 -> Sum10/2
  Sum16/1 -> Divide2/1
  Del Hr1/1 -> Product10/1
  Qi1/1 -> Product2/1
  Divide5/1 -> Sum10/3
  hA1/1 -> Product9/2
  Row c Cpc1/1 -> Product12/2
  Product10/1 -> Divide4/1
  Kd1/1 -> Sum15/2
  If1/1 -> Product2/2
  Divide3/1 -> Sum10/1
  Product6/1 -> Sum17/2
  Mf1/1 -> Product5/2
  Sum17/1 -> Integrator4/1
  Qt1/1 -> Sum8/1
  Kp1/1 -> Product6/1, Product10/2  "Kp"
  Tcf1/1 -> Sum13/2
  Integrator3/1 -> Kd1/1, Qt1/1  "M"
  Product9/1 -> Divide5/2, Divide7/1  "T hA(T-Tc)"
  Sum15/1 -> Integrator3/1
  Row Cp1/1 -> Product11/2, Divide4/2
  Sum11/1 -> Qt3/1
  Divide1/1 -> Sum15/1
  Product5/1 -> Sum16/2
  P1/1 -> Product6/2, Product10/3  "P"
  Vc1/1 -> Product12/1, Divide6/2
  Product2/1 -> Sum8/2
  V1/1 -> Product11/1, Divide3/2, Divide2/2, Divide1/2  "V"
  Sum8/1 -> Divide1/1
  Integrator4/1 -> Kp1/1, Ot2/1  "S"
  Divide6/1 -> Sum14/1
  Divide2/1 -> Sum17/1
  Divide7/1 -> Sum14/2
  Tf1/1 -> Sum11/2
  Qc1/1 -> Divide6/1
  Sum13/1 -> Qc1/1
  Product12/1 -> Divide7/2
  Integrator6/1 -> Sum13/1, Sum12/2  "TC"
  Qt3/1 -> Divide3/1
  Sum14/1 -> Sum6/2
  In1/1 -> Sum6/1
  Sum6/1 -> Integrator6/1

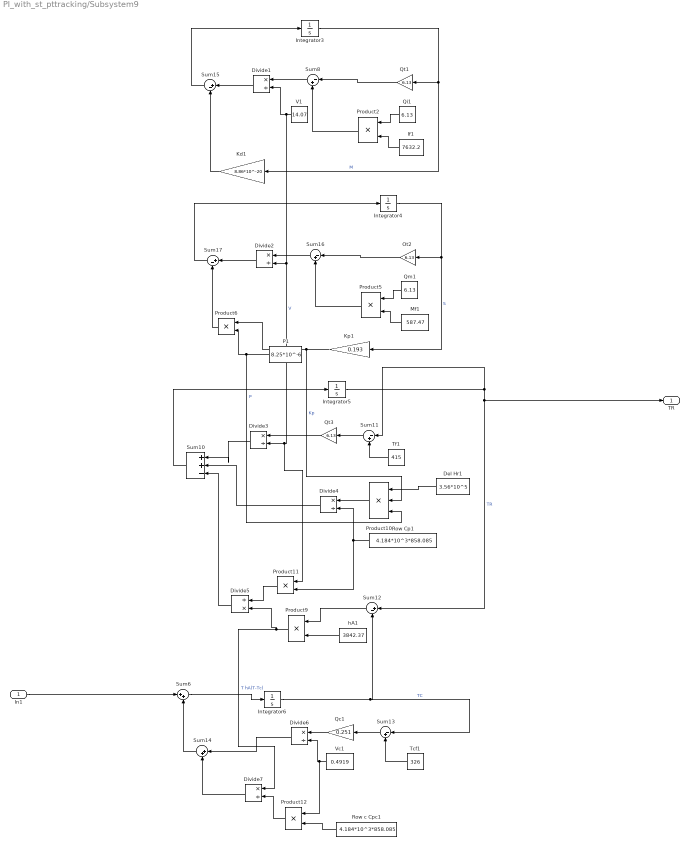
== system PI_with_st_pttracking/Subsystem9 ==
  In1 : Inport
  Del Hr1 : Constant  Value=3.56*10^5
  Divide{1..4,6..7} (6 alike) : Product  Inputs=*/
  Divide5 : Product  Inputs=/*
  If1 : Constant  Value=7632.2
  Integrator3 : Integrator  InitialCondition=7632.2
  Integrator4 : Integrator  InitialCondition=587.47
  Integrator5 : Integrator  InitialCondition=415
  Integrator6 : Integrator  InitialCondition=326
  Kd1 : Gain  Gain=8.86*10^-20
  Kp1 : Gain  Gain=0.193
  Mf1 : Constant  Value=587.47
  Ot2 : Gain  Gain=6.13
  P1 : Constant  Value=8.25*10^-6
  Product10 : Product  Inputs=3
  Product{2,5..6,9,11..12} (6 alike) : Product
  Qc1 : Gain  Gain=0.251
  Qi1 : Constant  Value=6.13
  Qm1 : Constant  Value=6.13
  Qt1 : Gain  Gain=6.13
  Qt3 : Gain  Gain=6.13
  Row Cp1 : Constant  Value=4.184*10^3*858.085
  Row c Cpc1 : Constant  Value=4.184*10^3*858.085
  Sum10 : Sum  Inputs=|++-
  Sum{8,11,13,16} (4 alike) : Sum  Inputs=|-+
  Sum12 : Sum  Inputs=|+-
  Sum14 : Sum  Inputs=|++
  Sum15 : Sum  Inputs=|+-
  Sum17 : Sum  Inputs=|+-
  Sum6 : Sum  Inputs=|++
  Tcf1 : Constant  Value=326
  Tf1 : Constant  Value=415
  V1 : Constant  Value=14.07
  Vc1 : Constant  Value=0.4919
  hA1 : Constant  Value=3842.37
  TR : Outport
  wires:
  Qm1/1 -> Product5/1
  Sum12/1 -> Product9/1
  Sum10/1 -> Integrator5/1
  Integrator5/1 -> TR/1, Sum12/1, Sum11/1  "TR"
  Ot2/1 -> Sum16/1
  Product11/1 -> Divide5/1
  Divide4/1 -> Sum10/2
  Sum16/1 -> Divide2/1
  Del Hr1/1 -> Product10/1
  Qi1/1 -> Product2/1
  Divide5/1 -> Sum10/3
  hA1/1 -> Product9/2
  Row c Cpc1/1 -> Product12/2
  Product10/1 -> Divide4/1
  Kd1/1 -> Sum15/2
  If1/1 -> Product2/2
  Divide3/1 -> Sum10/1
  Product6/1 -> Sum17/2
  Mf1/1 -> Product5/2
  Sum17/1 -> Integrator4/1
  Qt1/1 -> Sum8/1
  Kp1/1 -> Product6/1, Product10/2  "Kp"
  Tcf1/1 -> Sum13/2
  Integrator3/1 -> Kd1/1, Qt1/1  "M"
  Product9/1 -> Divide5/2, Divide7/1  "T hA(T-Tc)"
  Sum15/1 -> Integrator3/1
  Row Cp1/1 -> Product11/2, Divide4/2
  Sum11/1 -> Qt3/1
  Divide1/1 -> Sum15/1
  Product5/1 -> Sum16/2
  P1/1 -> Product6/2, Product10/3  "P"
  Vc1/1 -> Product12/1, Divide6/2
  Product2/1 -> Sum8/2
  V1/1 -> Product11/1, Divide3/2, Divide2/2, Divide1/2  "V"
  Sum8/1 -> Divide1/1
  Integrator4/1 -> Kp1/1, Ot2/1  "S"
  Divide6/1 -> Sum14/1
  Divide2/1 -> Sum17/1
  Divide7/1 -> Sum14/2
  Tf1/1 -> Sum11/2
  Qc1/1 -> Divide6/1
  Sum13/1 -> Qc1/1
  Product12/1 -> Divide7/2
  Integrator6/1 -> Sum13/1, Sum12/2  "TC"
  Qt3/1 -> Divide3/1
  Sum14/1 -> Sum6/2
  In1/1 -> Sum6/1
  Sum6/1 -> Integrator6/1
